simulink model "lab3"  (R2019b)
settings: Solver=VariableStepAuto  StartTime=0.0  StopTime=100  RelTol=1e-3
InitFcn:
  | W_bits = 16;
  | F_bits = 16;
  | 
  | p = 1;
  | q = 2;
  | 
  | filename ='C:\Users\Louis\Desktop\SoC-FPGAs-II\Lab 3\green_day.wav';
  | 
  | [y,Fs] = audioread(filename);
  | 
  | input_signal = resample(y,p,q);
  | 
  | t = zeros(length(input_signal),1);
  | 
  | for i = 1:length(input_signal)
  |   t(i) = 1/Fs * i;
  | end
  | 
  | input_signal = [t input_signal];
StopFcn:
  | sound(out.output_signal);
settings Model: Creator=Louis  LastModifiedBy=Louis

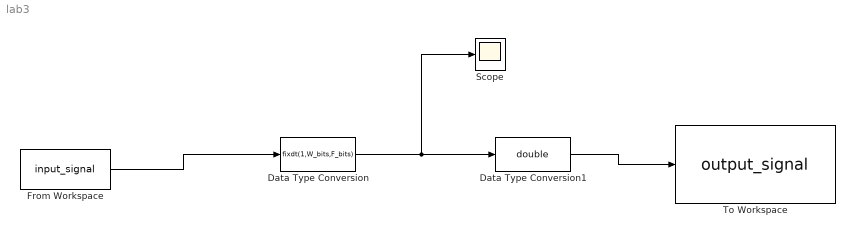
== system lab3 ==
  Data Type Conversion : DataTypeConversion  OutDataTypeStr=fixdt(1,W_bits,F_bits)  RndMeth=Convergent
  Data Type Conversion1 : DataTypeConversion  OutDataTypeStr=double
  From Workspace : FromWorkspace  VariableName=input_signal  SampleTime=0
  Scope : Scope
  To Workspace : ToWorkspace  VariableName=output_signal  SampleTime=-1
      settings: Save2DSignal=2-D array (concatenate along first dimension)
  wires:
  Data Type Conversion/1 -> Data Type Conversion1/1, Scope/1
  From Workspace/1 -> Data Type Conversion/1
  Data Type Conversion1/1 -> To Workspace/1
